simulink model "emABS_test1"  (R2024b)
settings: Solver=ode45  StartTime=0  StopTime=15  FixedStep=0.001  RelTol=1e-3  AbsTol=1e-6
undefined symbols (not defined in the file or in its folder): DiscIntNeverNeededParam
libraries: simulink x3, Solver_SF x1
settings Model: Creator=jhu  LastModifiedBy=황수빈
settings SolverCC: AutoScaleAbsTol=off  AlgebraicLoopSolver=TrustRegion
settings DataIOCC: SaveFormat=Array  SignalLoggingSaveFormat=ModelDataLogs  ReturnWorkspaceOutputs=off  SignalLoggingName=sigsOut
settings OptimizationCC: BlockReduction=off  BooleanDataType=off  ExpressionDepthLimit=2147483647  LifeSpan=inf
settings DebuggingCC: SaveWithParameterizedLinksMsg=none  UnderspecifiedInitializationDetection=Classic  MergeDetectMultiDrivingBlocksExec=none  SignalResolutionControl=TryResolveAllWithWarning  MultiTaskDSMMsg=warning  MultiTaskCondExecSysMsg=none  FcnCallInpInsideContextMsg=warning  UnconnectedInputMsg=warning  UnconnectedOutputMsg=warning  UnconnectedLineMsg=warning  StateNameClashWarn=warning  SFUnexpectedBacktrackingDiag=warning  SFNoUnconditionalDefaultTransitionDiag=warning  SFExecutionAtInitializationDiag=none  ArithmeticOperatorsInVariantConditions=warning
settings HardwareCC: ProdBitPerPointer=32  ProdBitPerSizeT=32  ProdBitPerPtrDiffT=32  ProdLargestAtomicFloat=None  ProdIntDivRoundTo=Undefined  ProdEndianess=Unspecified  ProdWordSize=32  ProdHWDeviceType=32-bit Generic  TargetUnknown=on
settings ModelReferenceCC: PropagateSignalLabelsOutOfModel=off
settings SFSimCC: SimUseLocalCustomCode=off  CustomCodeUndefinedFunction=UseInterfaceOnly
settings RTWCC: TemplateMakefile=grt_vc.tmf  RTWUseLocalCustomCode=off  GPUComputeCapability=3.5
settings CodeAppCC: StateflowObjectComments=on
settings GRTTargetCC: TargetFcnLib=ansi_tfl_tmw.mat  TargetLangStandard=C89/C90 (ANSI)  CombineOutputUpdateFcns=off  GRTInterface=on
settings ConfigComp: CovMetricSettings=dw  CovSaveCumulativeToWorkspaceVar=on  CovSaveSingleToWorkspaceVar=on  CovExternalEMLEnable=off

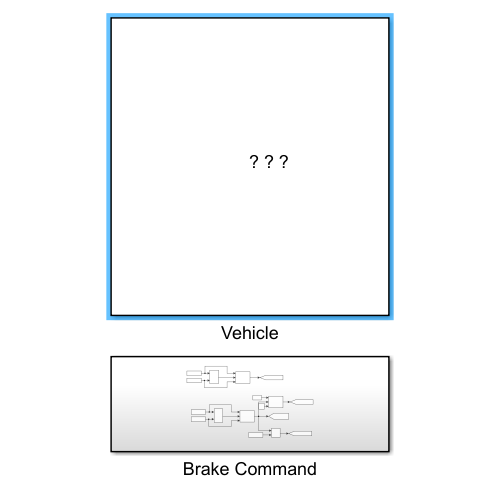
[thumbnail: Simulink's stored preview of the top-level diagram]
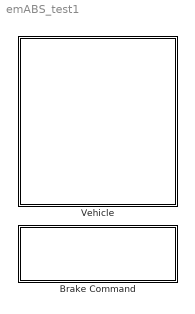
== system emABS_test1 ==
  Brake Command : Subsystem
  Vehicle : Subsystem
      mask Display: image('C:\Users\USER\Downloads\vehicle_icon.png'); % Use "Edit Image" on toolstrip to change.

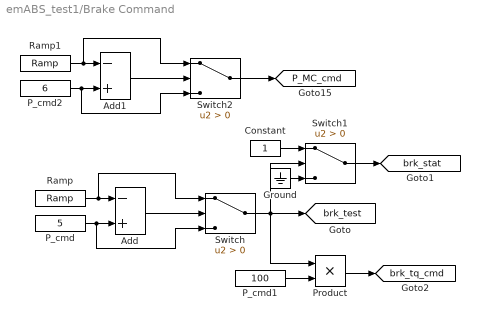
== system emABS_test1/Brake Command ==
  Add : Sum  Inputs=-+
  Add1 : Sum  Inputs=-+
  Constant : Constant
  Ground : Ground
  P_cmd : Constant  Value=5  SampleTime=0.01
  P_cmd1 : Constant  Value=100  SampleTime=0.01
  P_cmd2 : Constant  Value=6  SampleTime=0.01
  Product : Product
  Ramp : simulink/Sources/Ramp  slope=20  start=2  InitialOutput=0
  Ramp1 : simulink/Sources/Ramp  slope=20  start=2  InitialOutput=0
  Switch : Switch  Criteria=u2 > Threshold  SaturateOnIntegerOverflow=off  InputSameDT=off
  Switch1 : Switch  Criteria=u2 > Threshold  SaturateOnIntegerOverflow=off  InputSameDT=off
  Switch2 : Switch  Criteria=u2 > Threshold  SaturateOnIntegerOverflow=off  InputSameDT=off
  tag scope: P_MC_cmd=global, brk_stat=global, brk_test=global, brk_tq_cmd=global
  wires:
  P_cmd/1 -> Switch/3, Add/2
  Ramp/1 -> Switch/1, Add/1
  Add/1 -> Switch/2
  Switch/1 -> [brk_test], Product/1, Switch1/2
  Constant/1 -> Switch1/1
  Ground/1 -> Switch1/3
  Switch1/1 -> [brk_stat]
  P_cmd1/1 -> Product/2
  Product/1 -> [brk_tq_cmd]
  Add1/1 -> Switch2/2
  Ramp1/1 -> Switch2/1, Add1/1
  P_cmd2/1 -> Switch2/3, Add1/2
  Switch2/1 -> [P_MC_cmd]

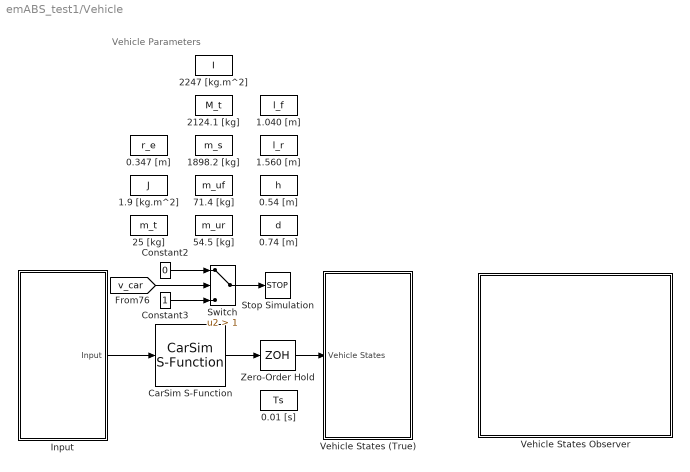
== system emABS_test1/Vehicle ==
  note: Vehicle Parameters
  0.01 [s] : DataStoreMemory  DataStoreName=Ts  WriteAfterWriteMsg=warning  InitialValue=0.01  ShowAdditionalParam=off  OutDataTypeStr=double
  0.347 [m] : DataStoreMemory  DataStoreName=r_e  WriteAfterWriteMsg=warning  InitialValue=0.347  ShowAdditionalParam=off  OutDataTypeStr=double
  0.54 [m] : DataStoreMemory  DataStoreName=h  WriteAfterWriteMsg=warning  InitialValue=0.54  ShowAdditionalParam=off  OutDataTypeStr=double
  0.74 [m] : DataStoreMemory  DataStoreName=d  WriteAfterWriteMsg=warning  InitialValue=0.819  ShowAdditionalParam=off  OutDataTypeStr=double
  1.040 [m] : DataStoreMemory  DataStoreName=l_f  WriteAfterWriteMsg=warning  InitialValue=1.44  ShowAdditionalParam=off  OutDataTypeStr=double
  1.560 [m] : DataStoreMemory  DataStoreName=l_r  WriteAfterWriteMsg=warning  InitialValue=1.56  ShowAdditionalParam=off  OutDataTypeStr=double
  1.9 [kg.m^2] : DataStoreMemory  DataStoreName=J  WriteAfterWriteMsg=warning  InitialValue=1.9  ShowAdditionalParam=off  OutDataTypeStr=double
  1898.2 [kg] : DataStoreMemory  DataStoreName=m_s  WriteAfterWriteMsg=warning  InitialValue=1908  ShowAdditionalParam=off  OutDataTypeStr=double
  2124.1 [kg] : DataStoreMemory  DataStoreName=M_t  WriteAfterWriteMsg=warning  InitialValue=2120  ShowAdditionalParam=off  OutDataTypeStr=double
  2247 [kg.m^2] : DataStoreMemory  DataStoreName=I  WriteAfterWriteMsg=warning  InitialValue=11460  ShowAdditionalParam=off  OutDataTypeStr=double
  25 [kg] : DataStoreMemory  DataStoreName=m_t  WriteAfterWriteMsg=warning  InitialValue=25  ShowAdditionalParam=off  OutDataTypeStr=double
  54.5 [kg] : DataStoreMemory  DataStoreName=m_ur  WriteAfterWriteMsg=warning  InitialValue=54.5  ShowAdditionalParam=off  OutDataTypeStr=double
  71.4 [kg] : DataStoreMemory  DataStoreName=m_uf  WriteAfterWriteMsg=warning  InitialValue=71.4  ShowAdditionalParam=off  OutDataTypeStr=double
  CarSim S-Function : Solver_SF/CarSim S-Function  Priority=1  SIMFILE=simfile.sim  Run_RTs=off  vs_state_ind=Run  StopMode_ind=Vehicle Model
  Constant2 : Constant  Value=0
  Constant3 : Constant
  Input : Subsystem
  Stop Simulation : Stop
  Switch : Switch  Criteria=u2 > Threshold  Threshold=1  SaturateOnIntegerOverflow=off  InputSameDT=off
  Vehicle States (True) : Subsystem
  Vehicle States Observer : Subsystem
  Zero-Order Hold : ZeroOrderHold  SampleTime=0.01
  wires:
  CarSim S-Function/1 -> Zero-Order Hold/1
  Zero-Order Hold/1 -> Vehicle States (True)/1(Vehicle States)
  Input/1(Input) -> CarSim S-Function/1
  Constant2/1 -> Switch/1
  [v_car] -> Switch/2
  Constant3/1 -> Switch/3
  Switch/1 -> Stop Simulation/1

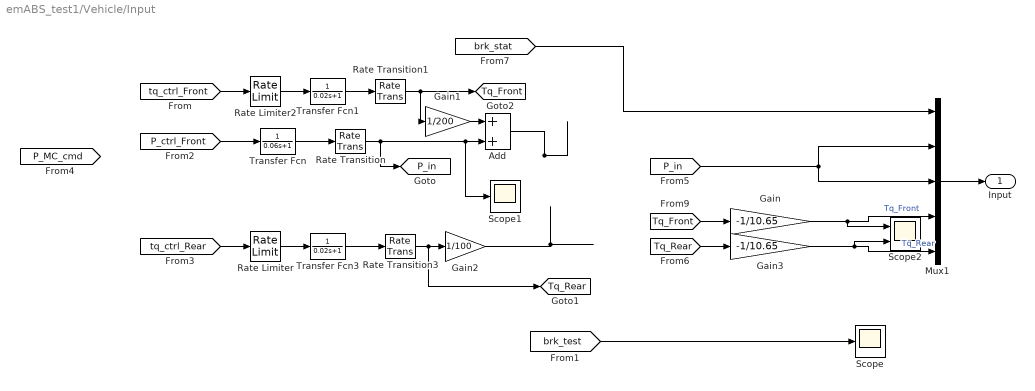
== system emABS_test1/Vehicle/Input ==
  Add : Sum
  Gain : Gain  Gain=-1/10.65
  Gain1 : Gain  Gain=1/200
  Gain2 : Gain  Gain=1/100
  Gain3 : Gain  Gain=-1/10.65
  Mux1 : Mux  Inputs=5
  Rate Limiter : RateLimiter  RisingSlewLimit=5000  FallingSlewLimit=-5000  SampleTimeMode=inherited
  Rate Limiter2 : RateLimiter  RisingSlewLimit=5000  FallingSlewLimit=-5000  SampleTimeMode=inherited
  Rate Transition : RateTransition  OutPortSampleTime=0.01
  Rate Transition1 : RateTransition  OutPortSampleTime=0.01
  Rate Transition3 : RateTransition  OutPortSampleTime=0.01
  Scope : Scope
  Scope1 : Scope
  Scope2 : Scope  NumInputPorts=2
  Transfer Fcn : TransferFcn  Denominator=[0.06 1]
  Transfer Fcn1 : TransferFcn  Denominator=[0.02 1]
  Transfer Fcn3 : TransferFcn  Denominator=[0.02 1]
  Input : Outport
  tag scope: P_in=global, Tq_Front=global, Tq_Rear=global
  wires:
  Transfer Fcn/1 -> Rate Transition/1
  [P_ctrl_Front] -> Transfer Fcn/1
  Mux1/1 -> Input/1
  [brk_stat] -> Mux1/1
  Gain2/1 -> ?
  Rate Transition/1 -> [P_in], Scope1/1, Add/2
  Transfer Fcn3/1 -> Rate Transition3/1
  Rate Transition3/1 -> [Tq_Rear], Gain2/1
  [tq_ctrl_Front] -> Rate Limiter2/1
  Transfer Fcn1/1 -> Rate Transition1/1
  Rate Transition1/1 -> [Tq_Front], Gain1/1
  Gain1/1 -> Add/1
  Add/1 -> ?
  Rate Limiter2/1 -> Transfer Fcn1/1
  [tq_ctrl_Rear] -> Rate Limiter/1
  Rate Limiter/1 -> Transfer Fcn3/1
  [brk_test] -> Scope/1
  [Tq_Rear] -> Gain3/1
  [Tq_Front] -> Gain/1
  Gain/1 -> Scope2/1, Mux1/4  "Tq_Front"
  Gain3/1 -> Scope2/2, Mux1/5  "Tq_Rear"
  [P_in] -> Mux1/3, Mux1/2

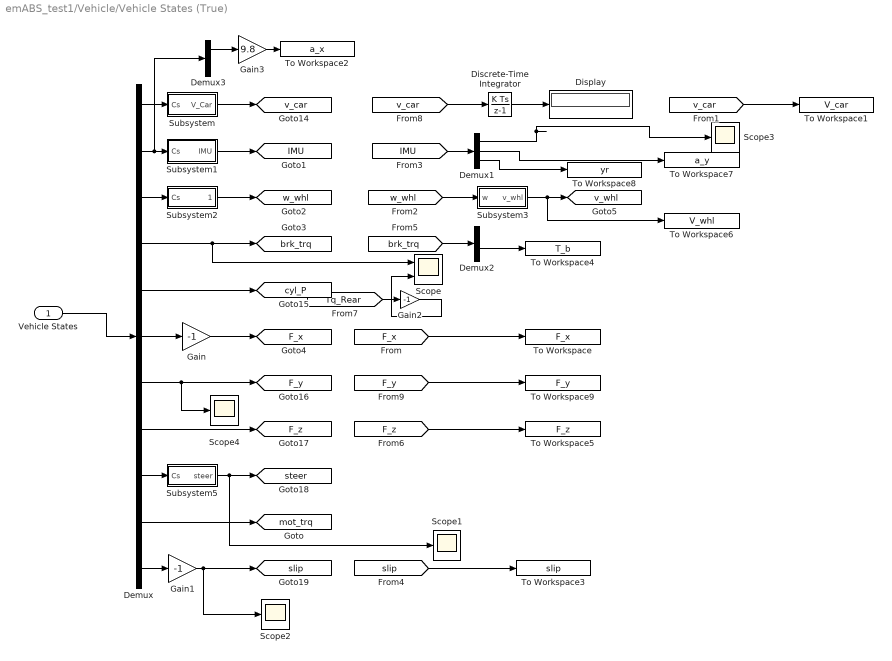
== system emABS_test1/Vehicle/Vehicle States (True) ==
  Vehicle States : Inport
  Demux : Demux  Outputs=[1 3 4 4 4 4 4 4 4 4 4]
  Demux1 : Demux  Outputs=3
  Demux2 : Demux
  Demux3 : Demux  Outputs=3
  Discrete-Time Integrator : DiscreteIntegrator  SampleTime=0.01  ICPrevOutput=DiscIntNeverNeededParam  ICPrevScaledInput=DiscIntNeverNeededParam
  Display : Display
      settings: Format=bank
  Gain : Gain  Gain=-1
  Gain1 : Gain  Gain=-1
  Gain2 : Gain  Gain=-1
  Gain3 : Gain  Gain=9.8
  Scope : Scope  NumInputPorts=2
  Scope{1..4} (4 alike) : Scope
  Subsystem : Subsystem
  Subsystem1 : Subsystem
  Subsystem2 : Subsystem
  Subsystem3 : Subsystem
  Subsystem5 : Subsystem
  To Workspace : ToWorkspace  VariableName=F_x  SaveFormat=Timeseries  SampleTime=-1
  To Workspace1 : ToWorkspace  VariableName=V_car  SaveFormat=Timeseries  SampleTime=-1
  To Workspace2 : ToWorkspace  VariableName=a_x  SaveFormat=Timeseries  SampleTime=-1
  To Workspace3 : ToWorkspace  VariableName=slip  SaveFormat=Timeseries  SampleTime=-1
  To Workspace4 : ToWorkspace  VariableName=T_b  SaveFormat=Timeseries  SampleTime=-1
  To Workspace5 : ToWorkspace  VariableName=F_z  SaveFormat=Timeseries  SampleTime=-1
  To Workspace6 : ToWorkspace  VariableName=V_whl  SaveFormat=Timeseries  SampleTime=-1
  To Workspace7 : ToWorkspace  VariableName=a_y  SaveFormat=Timeseries  SampleTime=-1
  To Workspace8 : ToWorkspace  VariableName=yr  SaveFormat=Timeseries  SampleTime=-1
  To Workspace9 : ToWorkspace  VariableName=F_y  SaveFormat=Timeseries  SampleTime=-1
  tag scope: F_x=global, F_y=global, F_z=global, IMU=global, brk_trq=global, cyl_P=global, mot_trq=global, slip=global, steer=global, v_car=global, v_whl=global, w_whl=global
  wires:
  Demux/6 -> Gain/1
  Demux/2 -> Demux3/1, Subsystem1/1(Cs)
  Subsystem/1(V_Car) -> [v_car]
  Demux/1 -> Subsystem/1(Cs)
  Demux/7 -> Scope4/1, [F_y]
  Subsystem1/1(IMU) -> [IMU]
  Vehicle States/1 -> Demux/1
  Demux/3 -> Subsystem2/1(Cs)
  Subsystem2/1(w_whl) -> [w_whl]
  Subsystem3/1(v_whl) -> To Workspace6/1, [v_whl]
  [w_whl] -> Subsystem3/1(w)
  Demux/4 -> Scope/1, [brk_trq]
  Demux/5 -> [cyl_P]
  Demux/8 -> [F_z]
  Demux/10 -> [mot_trq]
  Gain/1 -> [F_x]
  Demux/11 -> Gain1/1
  Subsystem5/1(steer) -> Scope1/1, [steer]
  Demux/9 -> Subsystem5/1(Cs)
  [v_car] -> Discrete-Time Integrator/1
  Discrete-Time Integrator/1 -> Display/1
  [F_x] -> To Workspace/1
  [v_car] -> To Workspace1/1
  [IMU] -> Demux1/1
  [slip] -> To Workspace3/1
  [brk_trq] -> Demux2/1
  Demux2/3 -> To Workspace4/1
  Gain1/1 -> Scope2/1, [slip]
  Demux1/1 -> Scope3/1
  [F_z] -> To Workspace5/1
  [Tq_Rear] -> Gain2/1
  Gain2/1 -> Scope/2
  Demux1/2 -> To Workspace7/1
  Demux1/3 -> To Workspace8/1
  [F_y] -> To Workspace9/1
  Demux3/1 -> Gain3/1
  Gain3/1 -> To Workspace2/1

== system emABS_test1/Vehicle/Vehicle States Observer ==
  Front/Rear Wheel Torque Control : Subsystem
  "Tire Force (Fx, Fy) Estimation" : Subsystem
  Vertical Tire Force (Fz) Estimation : Subsystem

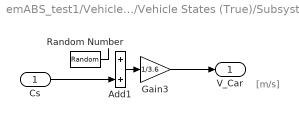
== system emABS_test1/Vehicle/Vehicle States (True)/Subsystem ==
  note: [m/s]
  Cs : Inport
  Add1 : Sum
  Gain3 : Gain  Gain=1/3.6
  Random Number : RandomNumber  Variance=0.0005  Seed=2  SampleTime=0.01
  V_Car : Outport
  wires:
  Random Number/1 -> ?
  Cs/1 -> Add1/2
  Add1/1 -> Gain3/1
  Gain3/1 -> V_Car/1

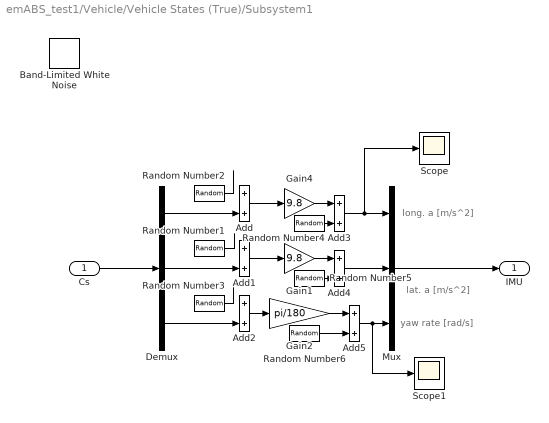
== system emABS_test1/Vehicle/Vehicle States (True)/Subsystem1 ==
  note: long. a [m/s^2]
  note: lat. a [m/s^2]
  note: yaw rate [rad/s]
  Cs : Inport
  Add{,1..5} (6 alike) : Sum
  Band-Limited White Noise : simulink/Sources/Band-Limited White Noise  Cov=[0.1]  Ts=0.1  seed=[23341]
  Demux : Demux  Outputs=3
  Gain1 : Gain  Gain=9.8
  Gain2 : Gain  Gain=pi/180
  Gain4 : Gain  Gain=9.8
  Mux : Mux  Inputs=3
  Random Number1 : RandomNumber  Variance=0.0001  Seed=2  SampleTime=0.01
  Random Number2 : RandomNumber  Variance=0.0001  Seed=1  SampleTime=0.01
  Random Number3 : RandomNumber  Variance=0.003  Seed=3  SampleTime=0.01
  Random Number4 : RandomNumber  Variance=0.01  Seed=1  SampleTime=0.01
  Random Number5 : RandomNumber  Variance=0.01  Seed=1000  SampleTime=0.01
  Random Number6 : RandomNumber  Variance=0.00001  Seed=3  SampleTime=0.01
  Scope : Scope
  Scope1 : Scope
  IMU : Outport
  wires:
  Random Number2/1 -> ?
  Gain4/1 -> Add3/1
  Cs/1 -> Demux/1
  Add/1 -> Gain4/1
  Demux/1 -> Add/2
  Demux/2 -> Add1/2
  Add1/1 -> Gain1/1
  Random Number1/1 -> ?
  Gain1/1 -> Add4/1
  Mux/1 -> IMU/1
  Demux/3 -> Add2/2
  Add2/1 -> Gain2/1
  Random Number3/1 -> ?
  Add3/1 -> Scope/1, Mux/1
  Random Number4/1 -> Add3/2
  Random Number5/1 -> Add4/2
  Add4/1 -> Mux/2
  Random Number6/1 -> Add5/2
  Gain2/1 -> Add5/1
  Add5/1 -> Scope1/1, Mux/3

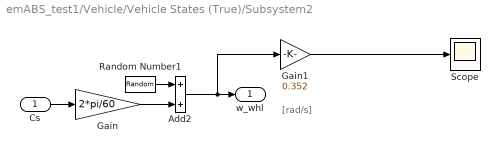
== system emABS_test1/Vehicle/Vehicle States (True)/Subsystem2 ==
  note: [rad/s]
  Cs : Inport
  Add2 : Sum
  Gain : Gain  Gain=2*pi/60
  Gain1 : Gain  Gain=0.352
  Random Number1 : RandomNumber  Variance=0.003  SampleTime=0.01
  Scope : Scope
  w_whl : Outport
  wires:
  Cs/1 -> Gain/1
  Add2/1 -> Gain1/1, w_whl/1
  Gain/1 -> Add2/2
  Random Number1/1 -> Add2/1
  Gain1/1 -> Scope/1

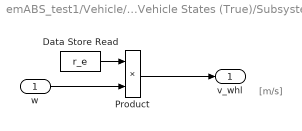
== system emABS_test1/Vehicle/Vehicle States (True)/Subsystem3 ==
  note: [m/s]
  w : Inport
  Data Store Read : DataStoreRead  DataStoreName=r_e  SampleTime=0.01  IndexOptions=Index vector (dialog)  Indices=1  OutputSizes=1
  Product : Product
  v_whl : Outport
  wires:
  w/1 -> Product/2
  Product/1 -> v_whl/1
  Data Store Read/1 -> Product/1

== system emABS_test1/Vehicle/Vehicle States (True)/Subsystem5 ==
  note: [rad]
  Cs : Inport
  Gain : Gain  Gain=pi/180
  steer : Outport
  wires:
  Cs/1 -> Gain/1
  Gain/1 -> steer/1

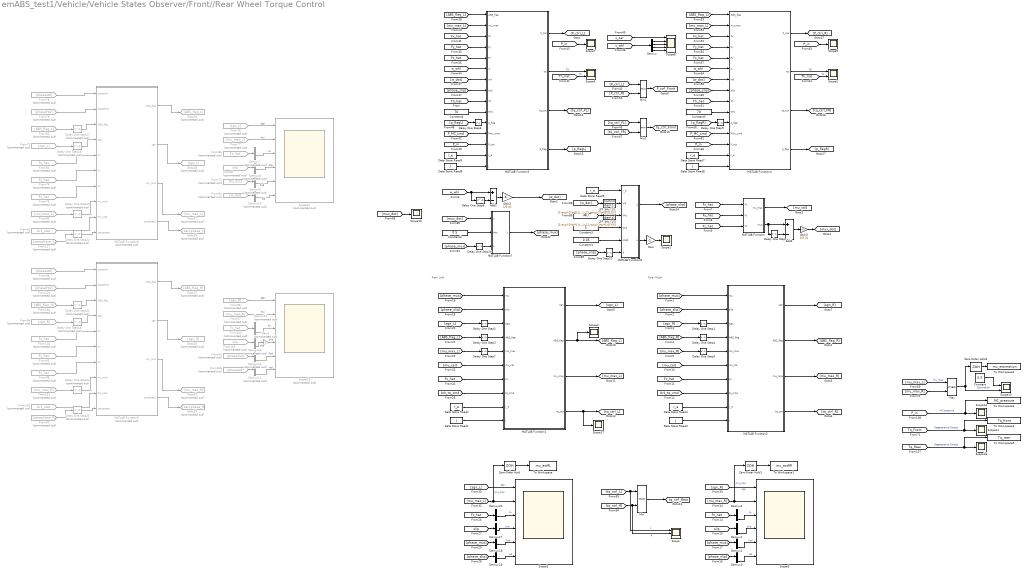
== system emABS_test1/Vehicle/Vehicle States Observer/Front//Rear Wheel Torque Control ==
  note: Rear Left
  note: Rear Right
  Add2 : Sum  Inputs=+-
  Add3 : Sum  Inputs=+-
  Constant : Constant  Value=0.5
  Constant1 : Constant  Value=0.05  SampleTime=0.01
  Constant2 : Constant  Value=0.5  SampleTime=0.01
  Constant3 : Constant  Value=5  SampleTime=0.01
  Constant4 : Constant  Value=70
  Constant5 : Constant  Value=70
  Data Store Read{1,3,6,8} (4 alike) : DataStoreRead  DataStoreName=J  SampleTime=0.01  IndexOptions=Index vector (dialog)  Indices=1  OutputSizes=1
  Data Store Read{2,4..5,7,9} (5 alike) : DataStoreRead  DataStoreName=r_e  SampleTime=0.01  IndexOptions=Index vector (dialog)  Indices=1  OutputSizes=1
  Delay One Step : Delay  DelayLength=1  InitialCondition=zeros(4,1)  SampleTime=0.01
  Delay One Step{1..9} (9 alike) : Delay  DelayLength=1  SampleTime=0.01
  Delay One Step{16..19,21,23..25} (8 alike) : Delay  Commented=on  DelayLength=1  InitialCondition=0  SampleTime=0.01
  Delay One Step20 : Delay  DelayLength=1  InitialCondition=zeros(4,1)  SampleTime=0.01
  Delay One Step22 : Delay  DelayLength=1  InitialCondition=zeros(4,1)  SampleTime=0.01
  Demux{,1..4,17..20} (9 alike) : Demux
  Demux{7..14} (8 alike) : Demux  Commented=on
  From100 : From  Commented=on  GotoTag=phaseFxd
  From101 : From  Commented=on  GotoTag=mu_max_R
  From102 : From  Commented=on  GotoTag=brk_stat  TagVisibility=global
  From{83..84,103,118} (4 alike) : From  Commented=on  GotoTag=Fx_hat  TagVisibility=global
  From104 : From  Commented=on  GotoTag=ABS_flag_R
  From105 : From  Commented=on  GotoTag=slip  TagVisibility=global
  From106 : From  Commented=on  GotoTag=phasewd
  From117 : From  Commented=on  GotoTag=zerophase_L
  From72 : From  Commented=on  GotoTag=sgn_L
  From73 : From  Commented=on  GotoTag=Fx_dot
  From74 : From  Commented=on  GotoTag=Fy_hat  TagVisibility=global
  From75 : From  Commented=on  GotoTag=Fz_hat  TagVisibility=global
  From76 : From  Commented=on  GotoTag=sgn_L
  From77 : From  Commented=on  GotoTag=mu_max_L
  From78 : From  Commented=on  GotoTag=phasewd
  From79 : From  Commented=on  GotoTag=phaseFxd
  From80 : From  Commented=on  GotoTag=mu_max_L
  From81 : From  Commented=on  GotoTag=brk_stat  TagVisibility=global
  From82 : From  Commented=on  GotoTag=ABS_flag_L
  From87 : From  Commented=on  GotoTag=slip  TagVisibility=global
  From90 : From  Commented=on  GotoTag=w_dot
  From92 : From  Commented=on  GotoTag=zerophase_R
  From93 : From  Commented=on  GotoTag=phaseFxd
  From94 : From  Commented=on  GotoTag=sgn_R
  From95 : From  Commented=on  GotoTag=Fy_hat  TagVisibility=global
  From96 : From  Commented=on  GotoTag=sgn_R
  From97 : From  Commented=on  GotoTag=mu_max_R
  From98 : From  Commented=on  GotoTag=Fz_hat  TagVisibility=global
  From99 : From  Commented=on  GotoTag=phasewd
  Gain : Gain  Gain=-1
  Gain2 : Gain  Gain=1/0.01
  Gain3 : Gain  Gain=1/0.01
  Gain5 : Gain  Commented=on  Gain=-1
  Goto18 : Goto  Commented=on  GotoTag=sgn_L
  Goto19 : Goto  Commented=on  GotoTag=ABS_flag_L
  Goto20 : Goto  Commented=on  GotoTag=sgn_R
  Goto21 : Goto  Commented=on  GotoTag=mu_max_L
  Goto23 : Goto  Commented=on  GotoTag=ABS_flag_R
  Goto25 : Goto  Commented=on  GotoTag=mu_max_R
  Goto28 : Goto  Commented=on  GotoTag=zerophase_L
  Goto29 : Goto  Commented=on  GotoTag=zerophase_R
  LPF 3Hz (1)1 : DiscreteFilter  Numerator=[1-exp(-2*pi*0.01*2)]  Denominator=[1 -exp(-2*pi*0.01*2)]  SampleTime=0.01
  LPF 3Hz (1)3 : DiscreteFilter  Numerator=[1-exp(-2*pi*0.01*3)]  Denominator=[1 -exp(-2*pi*0.01*3)]  SampleTime=0.01
  MATLAB Function : MATLAB Function  TreatAsAtomicUnit=on
  MATLAB Function1 : MATLAB Function  TreatAsAtomicUnit=on
  MATLAB Function2 : MATLAB Function  TreatAsAtomicUnit=on
  MATLAB Function3 : MATLAB Function  TreatAsAtomicUnit=on
  MATLAB Function4 : MATLAB Function  TreatAsAtomicUnit=on
  MATLAB Function6 : MATLAB Function  Commented=on  TreatAsAtomicUnit=on
  MATLAB Function7 : MATLAB Function  TreatAsAtomicUnit=on
  MATLAB Function8 : MATLAB Function  TreatAsAtomicUnit=on
  MATLAB Function9 : MATLAB Function  Commented=on  TreatAsAtomicUnit=on
  Max : MinMax  Function=max  Inputs=2
  Min : MinMax  Inputs=2
  Min1 : MinMax  Inputs=2
  Min2 : MinMax  Inputs=2
  Scope : Scope  NumInputPorts=3
  Scope{1,4,7,9..11,14,16..17} (9 alike) : Scope
  Scope12 : Scope  Commented=on  NumInputPorts=6
  Scope13 : Scope  Commented=on  NumInputPorts=6
  Scope15 : Scope  NumInputPorts=2
  Scope2 : Scope  NumInputPorts=2
  Scope3 : Scope  NumInputPorts=6
  Scope5 : Scope  NumInputPorts=6
  Scope6 : Scope  NumInputPorts=2
  Scope8 : Scope  NumInputPorts=5
  To Workspace : ToWorkspace  VariableName=mu_estRL  SaveFormat=Timeseries  SampleTime=-1
  To Workspace1 : ToWorkspace  VariableName=mu_estRR  SaveFormat=Timeseries  SampleTime=-1
  To Workspace2 : ToWorkspace  VariableName=mu_estimation  SaveFormat=Timeseries  SampleTime=-1
  To Workspace3 : ToWorkspace  VariableName=MC_pressure  SaveFormat=Timeseries  SampleTime=-1
  To Workspace4 : ToWorkspace  VariableName=Tq_front  SaveFormat=Timeseries  SampleTime=-1
  To Workspace5 : ToWorkspace  VariableName=Tq_rear  SaveFormat=Timeseries  SampleTime=-1
  Zero-Order Hold : ZeroOrderHold  SampleTime=0.01
  Zero-Order Hold1 : ZeroOrderHold  SampleTime=0.01
  Zero-Order Hold2 : ZeroOrderHold  SampleTime=0.01
  tag scope: P_ctrl_Front=global, tq_ctrl_Front=global, tq_ctrl_Rear=global
  wires:
  Delay One Step6/1 -> Add2/2
  [w_whl] -> Delay One Step6/1, Add2/1
  Add2/1 -> Gain2/1
  [tq_ctrl_R] -> Scope/2, Min/2  "R"
  [tq_ctrl_L] -> Scope/1, Min/1  "L"
  Min/1 -> [tq_ctrl_Rear]
  Gain2/1 -> [w_dot]
  From75/1 -> MATLAB Function6/7(Fz)
  From81/1 -> MATLAB Function6/9(brk_stat)
  MATLAB Function6/1(ABS_flag) -> Goto19/1
  From72/1 -> Delay One Step16/1
  From74/1 -> MATLAB Function6/6(Fy)
  From84/1 -> MATLAB Function6/5(Fx)
  From78/1 -> MATLAB Function6/1(phasewd)
  From82/1 -> Delay One Step17/1
  From80/1 -> Delay One Step19/1
  MATLAB Function6/3(mu_max) -> Goto21/1
  Delay One Step19/1 -> MATLAB Function6/8("mu_max ")
  Delay One Step17/1 -> MATLAB Function6/3("ABS_flag ")
  Delay One Step16/1 -> MATLAB Function6/4(sgn_)
  MATLAB Function6/2(sgn) -> Goto18/1
  [phase_mux] -> Delay One Step20/1
  Delay One Step22/1 -> MATLAB Function8/6("phase ")
  Constant3/1 -> MATLAB Function8/4(thrs)
  [phase_slip] -> Delay One Step22/1
  Delay One Step20/1 -> MATLAB Function7/3("phase ")
  Data Store Read9/1 -> MATLAB Function8/1(r_e)
  Constant2/1 -> MATLAB Function7/2(thrs)
  From79/1 -> MATLAB Function6/2(phaseFxd)
  From76/1 -> Scope12/1  "sgn"
  From77/1 -> Scope12/2  "mu"
  From83/1 -> Demux7/1
  From87/1 -> Demux8/1
  Demux7/3 -> Scope12/3  "Fx"
  Demux8/3 -> Scope12/4  "slip"
  From73/1 -> Demux9/1
  Demux9/3 -> Scope12/5  "Fxd"
  From90/1 -> Demux10/1
  Demux10/3 -> Scope12/6  "wd"
  From105/1 -> Demux13/1
  Demux11/4 -> Scope13/6  "wd"
  From103/1 -> Demux12/1
  From97/1 -> Scope13/2  "mu"
  Demux14/4 -> Scope13/5  "Fxd"
  From93/1 -> Demux14/1
  Demux12/4 -> Scope13/3  "Fx"
  Demux13/4 -> Gain5/1  "slip"
  From96/1 -> Scope13/1  "sgn"
  From106/1 -> Demux11/1
  MATLAB Function6/4(zerophase) -> Goto28/1
  Delay One Step24/1 -> MATLAB Function6/10("zerophase ")
  From117/1 -> Delay One Step24/1
  Gain5/1 -> Scope13/4  "slip"
  MATLAB Function7/1(phase) -> [phase_mux]
  MATLAB Function8/1(phase) -> [phase_slip]
  From104/1 -> Delay One Step21/1
  From95/1 -> MATLAB Function9/6(Fy)
  From99/1 -> MATLAB Function9/1(phasewd)
  Delay One Step25/1 -> MATLAB Function9/10("zerophase ")
  MATLAB Function9/4(zerophase) -> Goto29/1
  From92/1 -> Delay One Step25/1
  Delay One Step21/1 -> MATLAB Function9/3("ABS_flag ")
  From98/1 -> MATLAB Function9/7(Fz)
  From102/1 -> MATLAB Function9/9(brk_stat)
  From100/1 -> MATLAB Function9/2(phaseFxd)
  MATLAB Function9/2(sgn) -> Goto20/1
  From101/1 -> Delay One Step23/1
  Delay One Step18/1 -> MATLAB Function9/4(sgn_)
  From94/1 -> Delay One Step18/1
  MATLAB Function9/1(ABS_flag) -> Goto23/1
  MATLAB Function9/3(mu_max) -> Goto25/1
  Delay One Step23/1 -> MATLAB Function9/8("mu_max ")
  From118/1 -> MATLAB Function9/5(Fx)
  MATLAB Function8/2(u) -> Gain/1
  [Fx_hat] -> MATLAB Function/1(Fx)
  [Fy_hat] -> MATLAB Function/2(Fy)
  [Fz_hat] -> MATLAB Function/3(Fz)
  MATLAB Function/1(mu_max) -> [mu_cal]
  MATLAB Function/2(mux) -> Delay One Step/1, Add3/1
  Delay One Step/1 -> Add3/2
  Add3/1 -> Gain3/1
  Gain3/1 -> [mux_dot]
  [phase_mux] -> MATLAB Function1/1(mu)
  MATLAB Function1/1(sgn) -> [sgn_L]
  MATLAB Function1/2(ABS_flag) -> Scope4/1, [ABS_flag_L]
  MATLAB Function1/3(mu_max) -> [mu_max_L]
  MATLAB Function1/4(tq_out) -> Scope17/1, [tq_ctrl_L]
  [sgn_L] -> Delay One Step2/1
  Delay One Step2/1 -> MATLAB Function1/3(sgn_)
  [ABS_flag_L] -> Delay One Step3/1
  Delay One Step3/1 -> MATLAB Function1/4("ABS_flag ")
  [mu_max_L] -> Delay One Step7/1
  Delay One Step7/1 -> MATLAB Function1/5("mu_max ")
  [mu_cal] -> MATLAB Function1/6(mu_cal)
  [Fx_hat] -> MATLAB Function1/7(Fx)
  [brk_tq_cmd] -> MATLAB Function1/8(tq_cmd)
  Data Store Read2/1 -> MATLAB Function1/9(r_e)
  Data Store Read1/1 -> MATLAB Function1/10(J)
  [phase_mux] -> Demux18/1
  [phase_slip] -> Demux19/1
  [sgn_L] -> Scope3/1  "sgn"
  [Fx_hat] -> Demux20/1
  [slip] -> Demux17/1
  [mu_max_L] -> Zero-Order Hold/1, Scope3/2  "mu_max"
  Demux20/3 -> Scope3/3  "Fx"
  Demux18/3 -> Scope3/5  "Fxd"
  Demux19/3 -> Scope3/6  "wd"
  Demux17/3 -> Scope3/4  "slip"
  [mux_dot] -> MATLAB Function7/1(u)
  [w_dot] -> LPF 3Hz (1)1/1
  [IMU] -> LPF 3Hz (1)3/1
  LPF 3Hz (1)1/1 -> MATLAB Function8/2(wd)
  LPF 3Hz (1)3/1 -> MATLAB Function8/3(IMU)
  [phase_slip] -> MATLAB Function1/2(slip)
  Zero-Order Hold/1 -> To Workspace/1
  Delay One Step1/1 -> MATLAB Function2/3(sgn_)
  MATLAB Function2/4(tq_out) -> [tq_ctrl_R]
  Data Store Read4/1 -> MATLAB Function2/9(r_e)
  [ABS_flag_R] -> Delay One Step4/1
  [Fx_hat] -> MATLAB Function2/7(Fx)
  Delay One Step5/1 -> MATLAB Function2/5("mu_max ")
  MATLAB Function2/2(ABS_flag) -> [ABS_flag_R]
  [mu_max_R] -> Delay One Step5/1
  [mu_cal] -> MATLAB Function2/6(mu_cal)
  [sgn_R] -> Delay One Step1/1
  MATLAB Function2/1(sgn) -> [sgn_R]
  MATLAB Function2/3(mu_max) -> [mu_max_R]
  Data Store Read3/1 -> MATLAB Function2/10(J)
  [phase_mux] -> MATLAB Function2/1(mu)
  Delay One Step4/1 -> MATLAB Function2/4("ABS_flag ")
  [brk_tq_cmd] -> MATLAB Function2/8(tq_cmd)
  [phase_slip] -> MATLAB Function2/2(slip)
  [mu_max_R] -> Zero-Order Hold1/1, Scope5/2  "mu_max"
  Demux4/4 -> Scope5/3  "Fx"
  Demux3/4 -> Scope5/6  "wd"
  [Fx_hat] -> Demux4/1
  Demux2/4 -> Scope5/5  "Fxd"
  [phase_slip] -> Demux3/1
  Demux1/4 -> Scope5/4  "slip"
  [slip] -> Demux1/1
  [phase_mux] -> Demux2/1
  [sgn_R] -> Scope5/1  "sgn"
  Zero-Order Hold1/1 -> To Workspace1/1
  Constant1/1 -> MATLAB Function8/5(slipd)
  [Th_hat] -> MATLAB Function3/9(Th)
  [mu_max_L] -> MATLAB Function3/2(mu_max)
  [Fx_hat] -> MATLAB Function3/3(Fx)
  [Fy_hat] -> MATLAB Function3/4(Fy)
  [Fz_hat] -> MATLAB Function3/5(Fz)
  Data Store Read5/1 -> MATLAB Function3/14(r_e)
  MATLAB Function3/1(P_out) -> [P_ctrl_L]
  [ABS_flag_L] -> MATLAB Function3/1(ABS_flag)
  [P_ctrl_L] -> Min1/1
  Constant4/1 -> MATLAB Function3/10(thrs)
  MATLAB Function3/2(Td) -> Scope6/1  "Td"
  [Th_hat] -> Scope6/2  "Th"
  [P_MC_cmd] -> MATLAB Function3/12(Pmc_cmd)
  [P_in] -> MATLAB Function3/13("P_out ")
  [P_in] -> Scope7/1
  [w_whl] -> MATLAB Function3/6(w)
  [w_dot] -> MATLAB Function3/7(wd)
  Data Store Read6/1 -> MATLAB Function3/15(J)
  [tq_ctrl_FL] -> Min2/1
  [v_whl] -> Demux/1
  Demux/1 -> Scope8/2
  Demux/3 -> Scope8/4
  [phase_slip] -> MATLAB Function3/8(slip)
  MATLAB Function3/4(p_flag) -> [p_flagL]
  [p_flagL] -> Delay One Step8/1
  Delay One Step8/1 -> MATLAB Function3/11("p_flag ")
  [v_car] -> Scope8/1
  MATLAB Function3/3(tq_out) -> [tq_ctrl_FL]
  MATLAB Function4/3(tq_out) -> [tq_ctrl_FR]
  [P_in] -> Scope9/1
  [P_in] -> MATLAB Function4/13("P_out ")
  [w_whl] -> MATLAB Function4/6(w)
  Data Store Read8/1 -> MATLAB Function4/15(J)
  [Fx_hat] -> MATLAB Function4/3(Fx)
  [ABS_flag_L] -> MATLAB Function4/1(ABS_flag)
  [Fz_hat] -> MATLAB Function4/5(Fz)
  [w_dot] -> MATLAB Function4/7(wd)
  [Fy_hat] -> MATLAB Function4/4(Fy)
  Constant5/1 -> MATLAB Function4/10(thrs)
  [P_MC_cmd] -> MATLAB Function4/12(Pmc_cmd)
  Data Store Read7/1 -> MATLAB Function4/14(r_e)
  [Th_hat] -> MATLAB Function4/9(Th)
  MATLAB Function4/4(p_flag) -> [p_flagR]
  [mu_max_L] -> MATLAB Function4/2(mu_max)
  MATLAB Function4/1(P_out) -> [P_ctrl_R]
  Delay One Step9/1 -> MATLAB Function4/11("p_flag ")
  [phase_slip] -> MATLAB Function4/8(slip)
  [p_flagR] -> Delay One Step9/1
  [Th_hat] -> Scope2/2  "Th"
  MATLAB Function4/2(Td) -> Scope2/1  "Td"
  Demux/2 -> Scope8/3
  Demux/4 -> Scope8/5
  Min1/1 -> [P_ctrl_Front]
  [P_ctrl_R] -> Min1/2
  [tq_ctrl_FR] -> Min2/2
  Min2/1 -> [tq_ctrl_Front]
  Gain/1 -> Scope1/1
  [mux_dot] -> Scope10/1
  [mu_max_L] -> Max/1  "mu_max"
  [mu_max_R] -> Max/2
  Max/1 -> Scope15/2, Zero-Order Hold2/1  "Estimation"
  [P_in] -> To Workspace3/1, Scope14/1  "MC pressure"
  [Tq_Front] -> To Workspace4/1, Scope11/1  "Regenerative Torque"
  [Tq_Rear] -> To Workspace5/1, Scope16/1  "Regenerative Torque"
  Zero-Order Hold2/1 -> To Workspace2/1
  Constant/1 -> Scope15/1

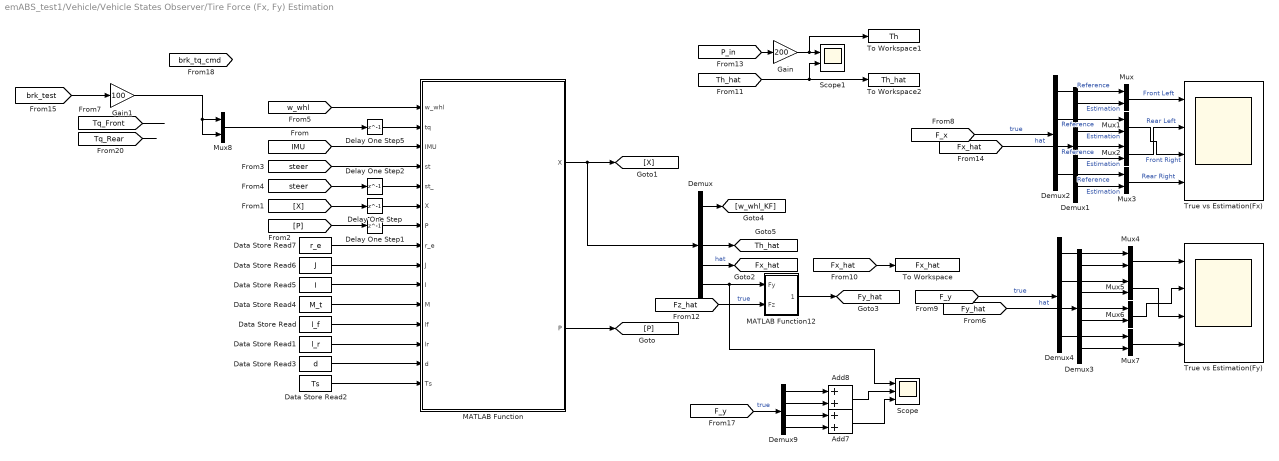
== system emABS_test1/Vehicle/Vehicle States Observer/Tire Force (Fx, Fy) Estimation ==
  Add7 : Sum
  Add8 : Sum
  Data Store Read : DataStoreRead  DataStoreName=l_f  SampleTime=0.01  IndexOptions=Index vector (dialog)  Indices=1  OutputSizes=1
  Data Store Read1 : DataStoreRead  DataStoreName=l_r  SampleTime=0.01  IndexOptions=Index vector (dialog)  Indices=1  OutputSizes=1
  Data Store Read2 : DataStoreRead  DataStoreName=Ts  SampleTime=0.01  IndexOptions=Index vector (dialog)  Indices=1  OutputSizes=1
  Data Store Read3 : DataStoreRead  DataStoreName=d  SampleTime=0.01  IndexOptions=Index vector (dialog)  Indices=1  OutputSizes=1
  Data Store Read4 : DataStoreRead  DataStoreName=M_t  SampleTime=0.01  IndexOptions=Index vector (dialog)  Indices=1  OutputSizes=1
  Data Store Read5 : DataStoreRead  DataStoreName=I  SampleTime=0.01  IndexOptions=Index vector (dialog)  Indices=1  OutputSizes=1
  Data Store Read6 : DataStoreRead  DataStoreName=J  SampleTime=0.01  IndexOptions=Index vector (dialog)  Indices=1  OutputSizes=1
  Data Store Read7 : DataStoreRead  DataStoreName=r_e  SampleTime=0.01  IndexOptions=Index vector (dialog)  Indices=1  OutputSizes=1
  Delay One Step : Delay  DelayLength=1  InitialCondition=[80 80 80 80 0 0 0 0 0 0 0 0]'  SampleTime=0.01
  Delay One Step1 : Delay  DelayLength=1  InitialCondition=diag([80 80 80 80 0 0 0 0 0 0 0 0])  SampleTime=0.01
  Delay One Step2 : Delay  DelayLength=1  InitialCondition=[0 0 0 0]'  SampleTime=0.01
  Delay One Step5 : Delay  DelayLength=1  InitialCondition=[0 0]'  SampleTime=0.01
  Demux : Demux  Outputs=[4 1 1 4 2]
  Demux{1..4,9} (5 alike) : Demux
  Gain : Gain  Gain=200
  Gain1 : Gain  Gain=100
  MATLAB Function : MATLAB Function  TreatAsAtomicUnit=on
  MATLAB Function12 : MATLAB Function  TreatAsAtomicUnit=on
  Mux{,1..8} (9 alike) : Mux  Inputs=2
  Scope : Scope  NumInputPorts=3
  Scope1 : Scope  NumInputPorts=2
  To Workspace : ToWorkspace  VariableName=Fx_hat  SaveFormat=Timeseries  SampleTime=-1
  To Workspace1 : ToWorkspace  VariableName=Th  SaveFormat=Timeseries  SampleTime=-1
  To Workspace2 : ToWorkspace  VariableName=Th_hat  SaveFormat=Timeseries  SampleTime=-1
  True vs Estimation(Fx) : Scope  NumInputPorts=4
  True vs Estimation(Fy) : Scope  NumInputPorts=4
  tag scope: Fx_hat=global, Fy_hat=global, Th_hat=global
  wires:
  Data Store Read/1 -> MATLAB Function/12(lf)
  Data Store Read1/1 -> MATLAB Function/13(lr)
  Data Store Read2/1 -> MATLAB Function/15(Ts)
  Data Store Read3/1 -> MATLAB Function/14(d)
  Data Store Read4/1 -> MATLAB Function/11(M)
  Data Store Read5/1 -> MATLAB Function/10(I)
  Data Store Read6/1 -> MATLAB Function/9(J)
  Data Store Read7/1 -> MATLAB Function/8(r_e)
  MATLAB Function/2(P) -> [P]
  MATLAB Function/1(X) -> Demux/1, [X]
  [X] -> Delay One Step/1
  Delay One Step/1 -> MATLAB Function/6("X ")
  [P] -> Delay One Step1/1
  Delay One Step1/1 -> MATLAB Function/7("P ")
  [steer] -> MATLAB Function/4(st)
  [steer] -> Delay One Step2/1
  Delay One Step2/1 -> MATLAB Function/5(st_)
  [w_whl] -> MATLAB Function/1(w_whl)
  Mux2/1 -> True vs Estimation(Fx)/2  "Rear Left"
  Mux3/1 -> True vs Estimation(Fx)/4  "Rear Right"
  Demux1/3 -> Mux2/2  "Estimation"
  Mux/1 -> True vs Estimation(Fx)/1  "Front Left"
  [Fx_hat] -> Demux1/1  "hat"
  Demux1/4 -> Mux3/2  "Estimation"
  Demux2/4 -> Mux3/1  "Reference"
  Demux1/2 -> Mux1/2  "Estimation"
  Demux1/1 -> Mux/2  "Estimation"
  Demux2/1 -> Mux/1  "Reference"
  Demux2/3 -> Mux2/1  "Reference"
  Mux1/1 -> True vs Estimation(Fx)/3  "Front Right"
  Demux2/2 -> Mux1/1  "Reference"
  [F_x] -> Demux2/1  "true"
  Mux8/1 -> Delay One Step5/1
  [Fz_hat] -> MATLAB Function12/2(Fz)  "true"
  Demux/4 -> [Fx_hat]  "hat"
  Demux/5 -> Scope/1, MATLAB Function12/1(Fy)
  MATLAB Function12/1(Fyhat) -> [Fy_hat]
  Demux4/1 -> Mux4/1
  Demux4/2 -> Mux5/1
  Demux3/4 -> Mux7/2
  Demux3/2 -> Mux5/2
  Demux3/1 -> Mux4/2
  Demux4/3 -> Mux6/1
  Demux4/4 -> Mux7/1
  Mux7/1 -> True vs Estimation(Fy)/4
  Mux6/1 -> True vs Estimation(Fy)/2
  Demux3/3 -> Mux6/2
  [F_y] -> Demux4/1  "true"
  Mux5/1 -> True vs Estimation(Fy)/3
  Mux4/1 -> True vs Estimation(Fy)/1
  [Fy_hat] -> Demux3/1  "hat"
  Demux/1 -> [w_whl_KF]
  [F_y] -> Demux9/1  "true"
  Demux9/4 -> Add7/2
  Demux9/3 -> Add7/1
  Demux9/1 -> Add8/1
  Demux9/2 -> Add8/2
  Add8/1 -> Scope/2
  Add7/1 -> Scope/3
  [IMU] -> MATLAB Function/3(IMU)
  Demux/3 -> [Th_hat]
  Delay One Step5/1 -> MATLAB Function/2(tq)
  [Fx_hat] -> To Workspace/1
  [P_in] -> Gain/1
  Gain/1 -> To Workspace1/1, Scope1/1
  [Th_hat] -> To Workspace2/1, Scope1/2
  [Tq_Front] -> ?
  [Tq_Rear] -> ?
  [brk_test] -> Gain1/1
  Gain1/1 -> Mux8/2, Mux8/1

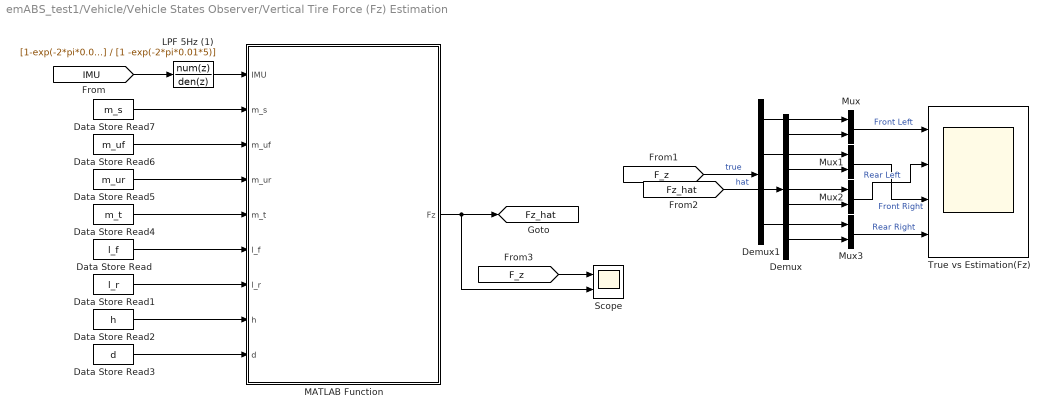
== system emABS_test1/Vehicle/Vehicle States Observer/Vertical Tire Force (Fz) Estimation ==
  Data Store Read : DataStoreRead  DataStoreName=l_f  SampleTime=0.01  IndexOptions=Index vector (dialog)  Indices=1  OutputSizes=1
  Data Store Read1 : DataStoreRead  DataStoreName=l_r  SampleTime=0.01  IndexOptions=Index vector (dialog)  Indices=1  OutputSizes=1
  Data Store Read2 : DataStoreRead  DataStoreName=h  SampleTime=0.01  IndexOptions=Index vector (dialog)  Indices=1  OutputSizes=1
  Data Store Read3 : DataStoreRead  DataStoreName=d  SampleTime=0.01  IndexOptions=Index vector (dialog)  Indices=1  OutputSizes=1
  Data Store Read4 : DataStoreRead  DataStoreName=m_t  SampleTime=0.01  IndexOptions=Index vector (dialog)  Indices=1  OutputSizes=1
  Data Store Read5 : DataStoreRead  DataStoreName=m_ur  SampleTime=0.01  IndexOptions=Index vector (dialog)  Indices=1  OutputSizes=1
  Data Store Read6 : DataStoreRead  DataStoreName=m_uf  SampleTime=0.01  IndexOptions=Index vector (dialog)  Indices=1  OutputSizes=1
  Data Store Read7 : DataStoreRead  DataStoreName=m_s  SampleTime=0.01  IndexOptions=Index vector (dialog)  Indices=1  OutputSizes=1
  Demux : Demux
  Demux1 : Demux
  LPF 5Hz (1) : DiscreteFilter  Numerator=[1-exp(-2*pi*0.01*5)]  Denominator=[1 -exp(-2*pi*0.01*5)]  SampleTime=0.01
  MATLAB Function : MATLAB Function  TreatAsAtomicUnit=on
  Mux{,1..3} (4 alike) : Mux  Inputs=2
  Scope : Scope  NumInputPorts=2
  True vs Estimation(Fz) : Scope  NumInputPorts=4
  tag scope: Fz_hat=global
  wires:
  Data Store Read/1 -> MATLAB Function/6(l_f)
  Data Store Read1/1 -> MATLAB Function/7(l_r)
  Data Store Read2/1 -> MATLAB Function/8(h)
  Data Store Read3/1 -> MATLAB Function/9(d)
  Data Store Read4/1 -> MATLAB Function/5(m_t)
  Data Store Read5/1 -> MATLAB Function/4(m_ur)
  Data Store Read6/1 -> MATLAB Function/3(m_uf)
  Data Store Read7/1 -> MATLAB Function/2(m_s)
  MATLAB Function/1(Fz) -> Scope/2, [Fz_hat]
  [F_z] -> Scope/1
  [Fz_hat] -> Demux/1  "hat"
  [F_z] -> Demux1/1  "true"
  Demux1/1 -> Mux/1
  Demux/1 -> Mux/2
  Demux1/2 -> Mux1/1
  Demux/2 -> Mux1/2
  Demux1/3 -> Mux2/1
  Demux/3 -> Mux2/2
  Demux1/4 -> Mux3/1
  Demux/4 -> Mux3/2
  [IMU] -> LPF 5Hz (1)/1
  LPF 5Hz (1)/1 -> MATLAB Function/1(IMU)
  Mux3/1 -> True vs Estimation(Fz)/4  "Rear Right"
  Mux1/1 -> True vs Estimation(Fz)/3  "Front Right"
  Mux/1 -> True vs Estimation(Fz)/1  "Front Left"
  Mux2/1 -> True vs Estimation(Fz)/2  "Rear Left"

== matlab function emABS_test1/Vehicle/Vehicle States Observer/Vertical Tire Force (Fz) Estimation/MATLAB Function ==
  data: IMU input; m_s input; m_uf input; m_ur input; m_t input; l_f input; l_r input; h input; d input; Fz output
function Fz = fcn(IMU, m_s, m_uf, m_ur, m_t, l_f, l_r, h, d)

a = [9.8 IMU(1) IMU(2)]';

L = l_f+l_r;
Mz = [l_r/(2*L)*m_s+1/2*m_uf+m_t -h/(2*L)*m_s -h*l_r/(2*d*L)*m_s;
     l_r/(2*L)*m_s+1/2*m_uf+m_t -h/(2*L)*m_s h*l_r/(2*d*L)*m_s;
     l_f/(2*L)*m_s+1/2*m_ur+m_t h/(2*L)*m_s -h*l_f/(2*d*L)*m_s;
     l_f/(2*L)*m_s+1/2*m_ur+m_t h/(2*L)*m_s h*l_f/(2*d*L)*m_s];

Fz = Mz*a;

== matlab function emABS_test1/Vehicle/Vehicle States Observer/Tire Force (Fx, Fy) Estimation/MATLAB Function ==
  data: w_whl input; tq input; IMU input; st input; st_ input; X input; P input; X output; P output; r_e input; J input; I input; M input; lf input; lr input; d input; Ts input
function [X,P]  = fcn(w_whl,tq,IMU,st,st_,X,P,r_e,J,I,M,lf,lr,d,Ts)

delta_ = (st_(1)+st_(2))/2;
delta = (st(1)+st(2))/2;

%X = [w_FL w_FR w_RL w_RR r tq_h Fx_FL Fx_FR Fx_RL Fx_RR Fy_F Fy_R]
Q = diag([0.001 0.001 0.0002 0.0002 0.000001 100 1000 1000 50 50 1000 1000]);

Z = [w_whl(1) w_whl(2) w_whl(3) w_whl(4) IMU(3) IMU(1) IMU(2)]';
R = diag([0.0002 0.0002 0.0002 0.0002 0.000001 0.001 0.001]);

U = [tq(1) tq(2)]';

F = eye(12) + Ts*...
    [0 0 0 0 0 -1/J r_e/J 0 0 0 0 0;
     0 0 0 0 0 -1/J 0 r_e/J 0 0 0 0;
     0 0 0 0 0 0 0 0 r_e/J 0 0 0;
     0 0 0 0 0 0 0 0 0 r_e/J 0 0;
     0 0 0 0 0 0 -lf/I*sin(st_(1))+d/I*cos(st_(1)) -lf/I*sin(st_(2))-d/I*cos(st_(2)) d/I -d/I lf/I*cos(delta_) -lr/I;
     zeros(7,12)];

G = Ts/J*[-1 0; -1 0; 0 -1; 0 -1;zeros(8,2)];

H = [eye(5) zeros(5,7);
     zeros(1,6) -cos(st(1))/M -cos(st(2))/M -1/M -1/M -sin(delta)/M 0;
     zeros(1,6) -sin(st(1))/M -sin(st(2))/M 0 0 cos(delta)/M 1/M];

Xm = F*X + G*U;
Pm = F*P*F' + Q;
K = Pm*H'/(H*Pm*H'+R);
X = Xm + K*(Z-H*Xm);
P = (eye(12)-K*H)*Pm;

end

== matlab function emABS_test1/Vehicle/Vehicle States Observer/Front//Rear Wheel Torque Control/MATLAB Function4 ==
  data: ABS_flag input; mu_max input; Fx input; Fy input; Fz input; w input; wd input; slip input; Th input; thrs input; p_flag input; Pmc_cmd input; P_out input; r_e input; J input; P_out output; Td output; tq_out output; p_flag output
function [P_out,Td,tq_out,p_flag]   = fcn(ABS_flag,mu_max,Fx,Fy,Fz,w,wd,slip,Th,thrs,p_flag,Pmc_cmd,P_out,r_e,J)

%% Front left
k = 2;
Fx = Fx(k); Fy = Fy(k);Fz = Fz(k); w_F = w(k); w_R = w(k+2); wd_R = wd(k+2); slip = slip(k);
%% Front Regen Control
if ABS_flag == 1
    if (w_F-w_R) > 0
        sgn = 1;
    else
        sgn = -1;
    end
    tq_out = max(0,r_e*Fx - J*wd_R -Th + 15*sgn);
    tq_out = min(tq_out,300);
else
    tq_out = 0;
    sgn = 0;
end
%% Brake Pressure Control
if ABS_flag == 1
    Td = 0.9*r_e*sqrt(abs((mu_max*Fz)^2-Fy^2));
    % if Th < (Td-thrs)
    %     P_out = P_out + 0.05;
    if tq_out == 0 && slip == 1 || p_flag == 1
        P_out = P_out - 2;
        if sgn == 1
            p_flag = 0;
        else
            p_flag = 1;
        end
            
    elseif Th > (Td+thrs)
        P_out = P_out - 1;
    elseif Th < (Td-thrs)
        P_out = P_out + 0.5;
    else
    end
else
    P_out = Pmc_cmd;
    Td = 0;
end
P_out = max(0,P_out);

% if Th < Td
%     sgn = 1;
% elseif Th 
%% Brake Pressure Control
% if ABS_flag == 1
%     tq_out = r_e*Fx + J/r_e*(mu_max*9.8) + 30*sgn;
%     mu_max = mu_cal;
% else
%     P_out = Pmc_cmd;
% end
%% ABS off
% if tq_out > tq_cmd
%     ABS_flag = 0;
% end

== matlab function emABS_test1/Vehicle/Vehicle States Observer/Front//Rear Wheel Torque Control/MATLAB Function6 ==
  data: ABS_flag output; sgn output; phasewd input; phaseFxd input; ABS_flag input; sgn_ input; Fx input; Fy input; Fz input; mu_max output; mu_max input; brk_stat input; zerophase input; zerophase output
function [ABS_flag,sgn,mu_max,zerophase]  = fcn(phasewd,phaseFxd,ABS_flag,sgn_,Fx,Fy,Fz,mu_max,brk_stat,zerophase)

% Rear Left
wd = phasewd(3); Fx = Fx(3); Fxd = phaseFxd(3); Fy = Fy(3); Fz = Fz(3);
if brk_stat == 1

    if wd == 0
        
        sgn = 0;
    else
        sgn = wd*Fxd;
    end

    if sgn-sgn_ < 0
        ABS_flag = 1;
    end
    if abs(sgn-sgn_) > 0 && ABS_flag == 1
        mu_max = sqrt(Fx^2+Fy^2)/Fz;
    end
else
    sgn = sgn_;
end

== matlab function emABS_test1/Vehicle/Vehicle States Observer/Front//Rear Wheel Torque Control/MATLAB Function7 ==
  data: u input; phase output; thrs input; phase input
function phase  = fcn(u,thrs,phase)
for i = 1:4
    if u(i) > thrs
        phase(i) = 1;
    elseif u(i) < -thrs
        phase(i) = -1;
    else
        phase(i) = 0;
    end
end

== matlab function emABS_test1/Vehicle/Vehicle States Observer/Tire Force (Fx, Fy) Estimation/MATLAB Function12 ==
  data: Fy input; Fz input; Fyhat output
function Fyhat = fcn(Fy, Fz)

kf = Fz(1)/Fz(2);
kr = Fz(3)/Fz(4);

Fylf = kf/(1+kf)*Fy(1);
Fyrf = 1/(1+kf)*Fy(1);
Fylr = kr/(1+kr)*Fy(2);
Fyrr = 1/(1+kr)*Fy(2);

Fyhat = [Fylf Fyrf Fylr Fyrr]';

== matlab function emABS_test1/Vehicle/Vehicle States Observer/Front//Rear Wheel Torque Control/MATLAB Function8 ==
  data: r_e input; wd input; IMU input; phase output; thrs input; slipd input; phase input; u output
function [phase,u]  = fcn(r_e,wd,IMU,thrs,slipd,phase)
u = r_e*wd -(1-slipd)*IMU(1);
for i = 1:4
    if u(i) > thrs
        phase(i) = -1;
    elseif u(i) < -thrs
        phase(i) = 1;
    else
        phase(i) = 0;
    end
end

== matlab function emABS_test1/Vehicle/Vehicle States Observer/Front//Rear Wheel Torque Control/MATLAB Function9 ==
  data: ABS_flag output; sgn output; phasewd input; phaseFxd input; ABS_flag input; sgn_ input; Fx input; Fy input; Fz input; mu_max output; mu_max input; brk_stat input; zerophase input; zerophase output
function [ABS_flag,sgn,mu_max,zerophase]  = fcn(phasewd,phaseFxd,ABS_flag,sgn_,Fx,Fy,Fz,mu_max,brk_stat,zerophase)

% Rear Left
wd = phasewd(4); Fx = Fx(4); Fxd = phaseFxd(4); Fy = Fy(4); Fz = Fz(4);
if brk_stat == 1

    if wd == 0
        sgn = sgn_;
    else
        sgn = wd*Fxd;
    end

    if sgn-sgn_ < 0
        ABS_flag = 1;
    end
    if abs(sgn-sgn_) > 0 && ABS_flag == 1
        mu_max = sqrt(Fx^2+Fy^2)/Fz;
    end
else
    sgn = sgn_;
end

== matlab function emABS_test1/Vehicle/Vehicle States Observer/Front//Rear Wheel Torque Control/MATLAB Function1 ==
  data: mu input; sgn output; slip input; sgn_ input; ABS_flag input; mu_max input; mu_cal input; Fx input; tq_cmd input; ABS_flag output; mu_max output; r_e input; J input; tq_out output
function [sgn,ABS_flag,mu_max,tq_out] = fcn(mu,slip,sgn_,ABS_flag,mu_max,mu_cal,Fx,tq_cmd,r_e,J)

%% Rear Left
mu = mu(3); slip = slip(3); mu_cal = mu_cal(3); Fx = Fx(3);
%% sgn
if mu == 0
    if slip == 1
        sgn = -1;
    else
        sgn = sgn_;
    end
elseif slip == 0
    sgn = sgn_;
else
    sgn = mu*slip;
end
%% ABS on & mu_max estimation
if slip == 1 && sgn_ == 1 && sgn == -1
    ABS_flag = 1;
    % mu_max = mu_cal;
else
end
%% Torque control
if ABS_flag == 1
    tq_out = r_e*Fx + J/r_e*(mu_max*9.8) + 23*sgn;
    if sgn == -1
        mu_max = mu_cal;
    end
else
    tq_out = tq_cmd;
end
%% ABS off
% if tq_out > tq_cmd
%     ABS_flag = 0;
% end

== matlab function emABS_test1/Vehicle/Vehicle States Observer/Front//Rear Wheel Torque Control/MATLAB Function ==
  data: Fx input; mu_max output; Fy input; Fz input; mux output
function [mu_max,mux] = fcn(Fx,Fy,Fz)

mu_max = sqrt(Fx.^2+Fy.^2)./Fz;
mux = sqrt(Fx.^2)./Fz;

== matlab function emABS_test1/Vehicle/Vehicle States Observer/Front//Rear Wheel Torque Control/MATLAB Function2 ==
  data: mu input; sgn output; slip input; sgn_ input; ABS_flag input; mu_max input; mu_cal input; Fx input; tq_cmd input; ABS_flag output; mu_max output; r_e input; J input; tq_out output
function [sgn,ABS_flag,mu_max,tq_out] = fcn(mu,slip,sgn_,ABS_flag,mu_max,mu_cal,Fx,tq_cmd,r_e,J)

%% Rear Left
mu = mu(4); slip = slip(4); mu_cal = mu_cal(4); Fx = Fx(4);
%% sgn
if mu == 0
    if slip == 1
        sgn = -1;
    else
        sgn = sgn_;
    end
elseif slip == 0
    sgn = sgn_;
else
    sgn = mu*slip;
end
%% ABS on & mu_max estimation
if slip == 1 && sgn_ == 1 && sgn == -1
    ABS_flag = 1;
    if sgn == -1
        mu_max = mu_cal;
    end
else
end
%% Torque control
if ABS_flag == 1
    tq_out = r_e*Fx + J/r_e*(mu_max*9.8) + 23*sgn;
    % mu_max = mu_cal;
else
    tq_out = tq_cmd;
end
%% ABS off
% if tq_out > tq_cmd
%     ABS_flag = 0;
% end

== matlab function emABS_test1/Vehicle/Vehicle States Observer/Front//Rear Wheel Torque Control/MATLAB Function3 ==
  data: ABS_flag input; mu_max input; Fx input; Fy input; Fz input; w input; wd input; slip input; Th input; thrs input; p_flag input; Pmc_cmd input; P_out input; r_e input; J input; P_out output; Td output; tq_out output; p_flag output
function [P_out,Td,tq_out,p_flag]   = fcn(ABS_flag,mu_max,Fx,Fy,Fz,w,wd,slip,Th,thrs,p_flag,Pmc_cmd,P_out,r_e,J)

%% Front left
k = 1;
Fx = Fx(k); Fy = Fy(k);Fz = Fz(k); w_F = w(k); w_R = w(k+2); wd_R = wd(k+2); slip = slip(k);
%% Front Regen Control
if ABS_flag == 1
    if (w_F-w_R) > 0
        sgn = 1;
    else
        sgn = -1;
    end
    tq_out = max(0,r_e*Fx - J*wd_R -Th + 15*sgn);
    tq_out = min(tq_out,300);
else
    tq_out = 0;
    sgn = 0;
end
%% Brake Pressure Control
if ABS_flag == 1
    Td = 0.9*r_e*sqrt(abs((mu_max*Fz)^2-Fy^2));
    % if Th < (Td-thrs)
    %     P_out = P_out + 0.05;
    if tq_out == 0 && slip == 1 || p_flag == 1
        P_out = P_out - 2;
        if sgn == 1
            p_flag = 0;
        else
            p_flag = 1;
        end
            
    elseif Th > (Td+thrs)
        P_out = P_out - 1;
    elseif Th < (Td-thrs)
        P_out = P_out + 0.5;
    else
    end
else
    P_out = Pmc_cmd;
    Td = 0;
end
P_out = max(0,P_out);

% if Th < Td
%     sgn = 1;
% elseif Th 
%% Brake Pressure Control
% if ABS_flag == 1
%     tq_out = r_e*Fx + J/r_e*(mu_max*9.8) + 30*sgn;
%     mu_max = mu_cal;
% else
%     P_out = Pmc_cmd;
% end
%% ABS off
% if tq_out > tq_cmd
%     ABS_flag = 0;
% end
